simulink model "Simulink_model"  (R2018b)
settings: Solver=VariableStepAuto  StartTime=0.0  StopTime=10.0  RelTol=1e-3
values from neighbouring files (symbols this model uses):
  c = zeros(4,12)    [Model.m]
  u_d = zeros(12,4)    [Model.m]
  x_d = zeros(12,12)    [Model.m]
undefined symbols (not defined in the file or in its folder): K
settings Model: Creator=Stefan's Laptop  LastModifiedBy=Stefan's Laptop

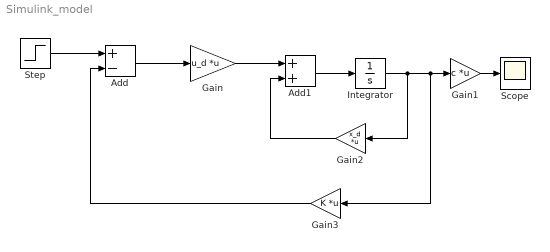
== system Simulink_model ==
  Add : Sum  Inputs=+-
  Add1 : Sum
  Gain : Gain  Gain=u_d  Multiplication=Matrix(K*u)
  Gain1 : Gain  Gain=c  Multiplication=Matrix(K*u)
  Gain2 : Gain  Gain=x_d  Multiplication=Matrix(K*u)
  Gain3 : Gain  Gain=K  Multiplication=Matrix(K*u)
  Integrator : Integrator
  Scope : Scope
  Step : Step  SampleTime=0
  wires:
  Step/1 -> Add/1
  Add/1 -> Gain/1
  Gain/1 -> Add1/1
  Add1/1 -> Integrator/1
  Integrator/1 -> Gain2/1, Gain3/1, Gain1/1
  Gain1/1 -> Scope/1
  Gain2/1 -> Add1/2
  Gain3/1 -> Add/2
